simulink model "single_vector"  (R2018b)
settings: Solver=ode1  StartTime=0.0  StopTime=0.7  FixedStep=1e-6  RelTol=1e-4
undefined symbols (not defined in the file): Ba, DiscIntNeverNeededParam, flux, Ki, Kp, L, R, states, Ts, v
libraries: powerlib x4
settings Model: SimulationMode=accelerator  ExtModeTrigMode=oneshot  ExtModeArmWhenConnect=off  ExtModeAutoUpdateStatusClock=off  Creator=Administrador  LastModifiedBy=123
settings DataIOCC: SaveFormat=Array  SignalLoggingSaveFormat=ModelDataLogs  SignalLoggingName=sigsOut
settings OptimizationCC: BlockReduction=off  BooleanDataType=off  ExpressionDepthLimit=2147483647  InitFltsAndDblsToZero=on  LifeSpan=inf
settings DebuggingCC: SaveWithParameterizedLinksMsg=none  UnderspecifiedInitializationDetection=Classic  MergeDetectMultiDrivingBlocksExec=none  SignalResolutionControl=TryResolveAllWithWarning  MultiTaskDSMMsg=warning  MultiTaskCondExecSysMsg=none  FcnCallInpInsideContextMsg=warning  StateNameClashWarn=warning  LibraryContextMissingDiagnostic=none  SFUnexpectedBacktrackingDiag=warning  SFNoUnconditionalDefaultTransitionDiag=warning  SFExecutionAtInitializationDiag=none
settings HardwareCC: ProdBitPerPointer=32  ProdBitPerSizeT=32  ProdBitPerPtrDiffT=32  ProdLargestAtomicFloat=None  ProdIntDivRoundTo=Undefined  ProdEndianess=Unspecified  ProdWordSize=32  ProdHWDeviceType=32-bit Generic  TargetUnknown=on
settings ModelReferenceCC: PropagateSignalLabelsOutOfModel=off
settings SFSimCC: SimUseLocalCustomCode=off
settings RTWCC: RTWUseLocalCustomCode=off
settings CodeAppCC: StateflowObjectComments=on
settings GRTTargetCC: TargetFcnLib=ansi_tfl_tmw.mat  TargetLangStandard=C89/C90 (ANSI)  GeneratePreprocessorConditionals=Disable all  CombineOutputUpdateFcns=off  GRTInterface=on
settings ConfigComp: CovMetricSettings=dw  CovHtmlReporting=on  CovSaveCumulativeToWorkspaceVar=on  CovSaveSingleToWorkspaceVar=on  CovExternalEMLEnable=off  CovSFcnEnable=off

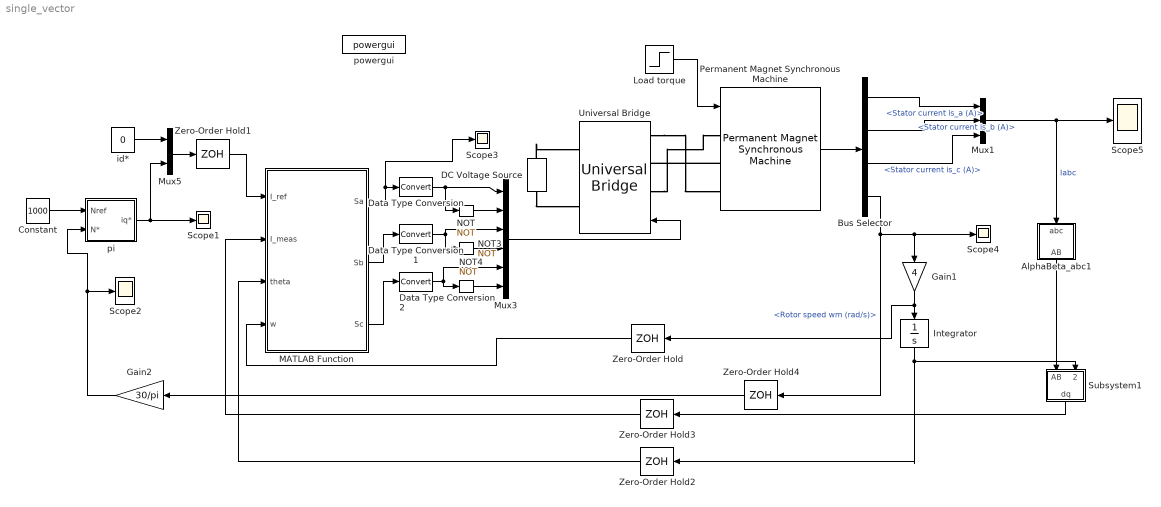
== system single_vector ==
  AlphaBeta_abc1 : Subsystem
  Bus Selector : BusSelector  OutputSignals=Stator current is_a (A),Stator current is_b (A),Stator current is_c (A),Rotor speed wm (rad/s)
  Constant : Constant  Value=1000
  DC Voltage Source : powerlib/Electrical Sources/DC Voltage Source  Amplitude=311  Measurements=None
      settings: SourceProductName=Simscape Electrical
  Data Type Conversion : DataTypeConversion
  Data Type Conversion1 : DataTypeConversion
  Data Type Conversion2 : DataTypeConversion
  Gain1 : Gain  Gain=4
  Gain2 : Gain  Gain=30/pi
  Integrator : Integrator
  Load torque : Step  Time=0.35  After=5  SampleTime=1e-6
  MATLAB Function : MATLAB Function  TreatAsAtomicUnit=on  SystemSampleTime=5e-6
  Mux1 : Mux  Inputs=3
  Mux3 : Mux  Inputs=6
  Mux5 : Mux  Inputs=2
  NOT : Logic  Operator=NOT  IconShape=distinctive  AllPortsSameDT=off  OutDataTypeStr=boolean
  NOT3 : Logic  Operator=NOT  IconShape=distinctive  AllPortsSameDT=off  OutDataTypeStr=boolean
  NOT4 : Logic  Operator=NOT  IconShape=distinctive  AllPortsSameDT=off  OutDataTypeStr=boolean
  Permanent Magnet Synchronous Machine : powerlib/Machines/Permanent Magnet Synchronous Machine  NbPhases=3  FluxDistribution=Sinusoidal  RotorType=Round  MechanicalLoad=Torque Tm  PresetModel=No  ShowDetailedParameters=on  MeasurementBus=off  Resistance=0.958  Inductance=8.5e-3  dqInductances=[5.25e-3,12e-3]  La=6e-3  MachineConstant=Flux linkage established by magnets (V.s)  Flux=0.1827  VoltageCst=132.5525  TorqueCst=1.0962  Flat=120  Mechanical=[0.003 0.008 4 0]  PolePairs=4  InitialConditions=[0,0, 0,0]  InitialConditions5ph=[0 0 0 0 0 0]  TsPowergui=0  TsBlock=-1  RefAngle=Aligned with phase A axis (original Park)
  Scope{1..5} (5 alike) : Scope
  Subsystem1 : Subsystem
  Universal Bridge : powerlib/Power Electronics/Universal Bridge  Arms=3  SnubberResistance=1e5  SnubberCapacitance=inf  Device=IGBT / Diodes  Ron=1e-3  Lon=0  ForwardVoltages="[  0  0  ]"  ForwardVoltage=0  GTOparameters=[ 10e-6 , 20e-6 ]  IGBTparameters=[ 1e-6 , 2e-6 ]  Measurements=None  Measurements_2=None  converterType=Rectifier
      settings: SourceProductName=Simscape Electrical
  Zero-Order Hold{,1..4} (5 alike) : ZeroOrderHold  SampleTime=5e-6
  id* : Constant  Value=0
  pi : Subsystem
  powergui : powerlib/powergui  Priority=1  SimulationMode=Discrete  SampleTime=1e-6  frequency=60  Iterations=50  frequencyindice=0  Pbase=100e6  ErrMax=1e-4  UnitsV=kV  UnitsW=MW  buscounter=0  FunctionMessages=off  echomessages=off  EnableUseOfTLC=off  CurrentSourceSwitches=off  DisableSnubberDevices=off  DisableRonSwitches=off  DisableVfSwitches=off  DisplayEquations=off  SolverType=Tustin  Interpol=off  ExternalGateDelay=off  methode=off  Ts=0  x0status=blocks  SPID=off  SwTol=0  HookPort=off  RestoreLinks=warning  ResistiveCurrentMeasurement=off  Frange=[0:2:500]  Ylog=off  Xlog=on  ShowGrid=off  save=off  variable=ZData  structure=ScopeData  ZoomFFT=off  StartTime=0.05  cycles=1  DisplayStyle=1  fundamental=50  FreqAxis=off  MaxFrequency=2000  frequencyindicesteady=1  RmsSteady=1  display=off
  wires:
  Mux1/1 -> Scope5/1, AlphaBeta_abc1/1(abc)  "Iabc"
  MATLAB Function/1(Sa) -> Scope3/1, Data Type Conversion/1
  NOT/1 -> Mux3/2
  MATLAB Function/2(Sb) -> Data Type Conversion1/1
  NOT3/1 -> Mux3/4
  MATLAB Function/3(Sc) -> Data Type Conversion2/1
  NOT4/1 -> Mux3/6
  Mux3/1 -> Universal Bridge/1
  Permanent Magnet Synchronous Machine/1 -> Bus Selector/1
  Bus Selector/1 -> Mux1/1  "<Stator current is_a (A)>"
  Bus Selector/2 -> Mux1/2  "<Stator current is_b (A)>"
  Bus Selector/3 -> Mux1/3  "<Stator current is_c (A)>"
  Constant/1 -> pi/1(Nref)
  Bus Selector/4 -> Gain1/1, Scope4/1, Zero-Order Hold4/1  "<Rotor speed wm (rad/s)>"
  AlphaBeta_abc1/1(AB) -> Subsystem1/1(AB)
  id*/1 -> Mux5/1
  pi/1(iq*) -> Scope1/1, Mux5/2
  Data Type Conversion/1 -> NOT/1, Mux3/1
  Data Type Conversion1/1 -> Mux3/3, NOT3/1
  Data Type Conversion2/1 -> Mux3/5, NOT4/1
  Mux5/1 -> Zero-Order Hold1/1
  Gain1/1 -> Zero-Order Hold/1, Integrator/1
  Integrator/1 -> Zero-Order Hold2/1, Subsystem1/2(theta)
  Load torque/1 -> Permanent Magnet Synchronous Machine/1
  Gain2/1 -> Scope2/1, pi/2(N*)
  Subsystem1/1(dq) -> Zero-Order Hold3/1
  Zero-Order Hold/1 -> MATLAB Function/4(w)
  Zero-Order Hold1/1 -> MATLAB Function/1(I_ref)
  Zero-Order Hold2/1 -> MATLAB Function/3(theta)
  Zero-Order Hold3/1 -> MATLAB Function/2(I_meas)
  Zero-Order Hold4/1 -> Gain2/1
  connections:
  DC Voltage Source/RConn1 -- Universal Bridge/RConn1
  DC Voltage Source/LConn1 -- Universal Bridge/RConn2
  Universal Bridge/LConn3 -- Permanent Magnet Synchronous Machine/LConn3
  Permanent Magnet Synchronous Machine/LConn2 -- Universal Bridge/LConn2
  Universal Bridge/LConn1 -- Permanent Magnet Synchronous Machine/LConn1

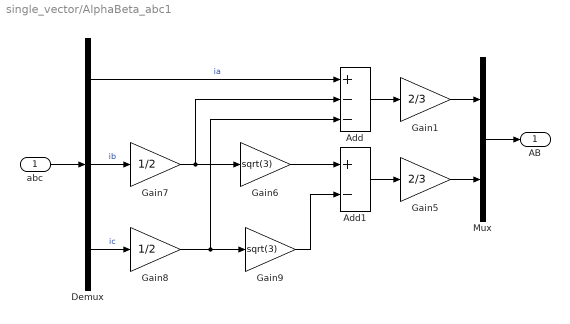
== system single_vector/AlphaBeta_abc1 ==
  abc : Inport
  Add : Sum  Inputs=+--
  Add1 : Sum  Inputs=+-
  Demux : Demux  Outputs=3
  Gain1 : Gain  Gain=2/3
  Gain5 : Gain  Gain=2/3
  Gain6 : Gain  Gain=sqrt(3)
  Gain7 : Gain  Gain=1/2
  Gain8 : Gain  Gain=1/2
  Gain9 : Gain  Gain=sqrt(3)
  Mux : Mux  Inputs=2
  AB : Outport
  wires:
  abc/1 -> Demux/1
  Demux/2 -> Gain7/1  "ib"
  Demux/3 -> Gain8/1  "ic"
  Add/1 -> Gain1/1
  Gain7/1 -> Gain6/1, Add/2
  Gain8/1 -> Gain9/1, Add/3
  Gain6/1 -> Add1/1
  Gain9/1 -> Add1/2
  Demux/1 -> Add/1  "ia"
  Add1/1 -> Gain5/1
  Gain1/1 -> Mux/1
  Gain5/1 -> Mux/2
  Mux/1 -> AB/1

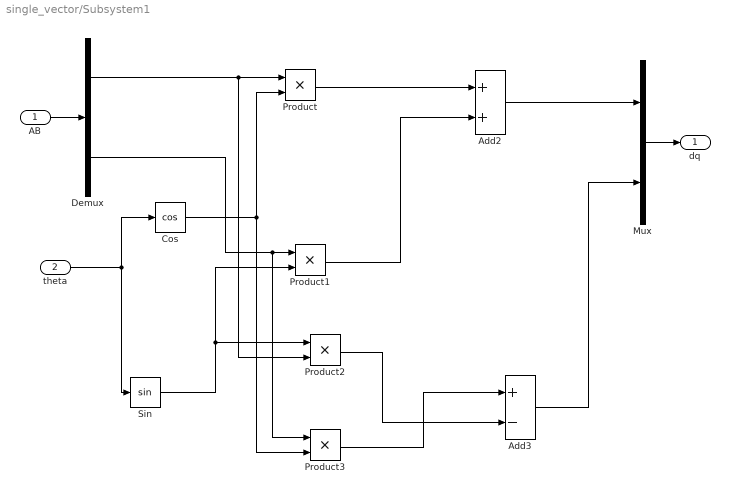
== system single_vector/Subsystem1 ==
  AB : Inport
  theta : Inport  Port=2
  Add2 : Sum
  Add3 : Sum  Inputs=+-
  Cos : Trigonometry  Operator=cos
  Demux : Demux  Outputs=2
  Mux : Mux  Inputs=2
  Product{,1..3} (4 alike) : Product
  Sin : Trigonometry
  dq : Outport
  wires:
  Product2/1 -> Add3/2
  Product/1 -> Add2/1
  theta/1 -> Sin/1, Cos/1
  Mux/1 -> dq/1
  AB/1 -> Demux/1
  Add3/1 -> Mux/2
  Add2/1 -> Mux/1
  Cos/1 -> Product3/2, Product/2
  Demux/2 -> Product1/1, Product3/1
  Demux/1 -> Product/1, Product2/2
  Product1/1 -> Add2/2
  Product3/1 -> Add3/1
  Sin/1 -> Product2/1, Product1/2

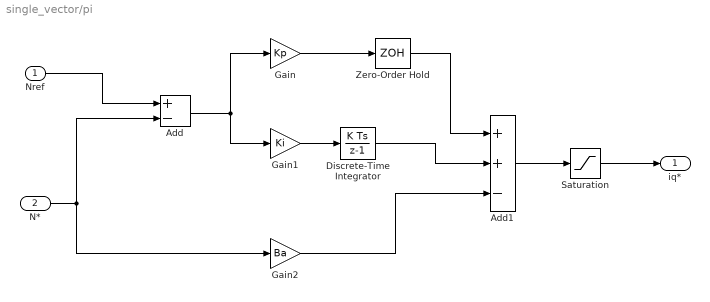
== system single_vector/pi ==
  Nref : Inport
  N* : Inport  Port=2
  Add : Sum  Inputs=+-
  Add1 : Sum  Inputs=++-
  Discrete-Time Integrator : DiscreteIntegrator  SampleTime=-1  ICPrevOutput=DiscIntNeverNeededParam  ICPrevScaledInput=DiscIntNeverNeededParam
  Gain : Gain  Gain=Kp
  Gain1 : Gain  Gain=Ki
  Gain2 : Gain  Gain=Ba
  Saturation : Saturate  UpperLimit=10  LowerLimit=-10
  Zero-Order Hold : ZeroOrderHold  SampleTime=-1
  iq* : Outport
  wires:
  Nref/1 -> Add/1
  N*/1 -> Gain2/1, Add/2
  Add/1 -> Gain1/1, Gain/1
  Gain/1 -> Zero-Order Hold/1
  Zero-Order Hold/1 -> Add1/1
  Gain1/1 -> Discrete-Time Integrator/1
  Discrete-Time Integrator/1 -> Add1/2
  Gain2/1 -> Add1/3
  Add1/1 -> Saturation/1
  Saturation/1 -> iq*/1

== matlab function single_vector/MATLAB Function ==
  data: I_ref input; Sa output; I_meas input; theta input; w input; Sb output; Sc output; R parameter; L parameter; Ts parameter; v parameter; states parameter; flux parameter
function [Sa,Sb,Sc] = control(I_ref,I_meas,theta,w,R, L, Ts, v, states, flux)

persistent x_old i_old 

if isempty(x_old), x_old = 1; end
if isempty(i_old), i_old = 0+1j*0; end
g = zeros(1,7);

ik_ref = I_ref(1) + 1j*I_ref(2);

ik = I_meas(1) + 1j*I_meas(2);
is = ik*exp(1j*theta);

% e = v(x_old) - L/Ts*is - (R - L/Ts)*i_old;
e = v(x_old) - R*(is+i_old)-L/Ts*(is-i_old);
en = e*exp(-1j*theta);

i_old = is;
for i = 1:7
    
    v_o1 = v(i)*exp(-1j*theta);
    
    % ik1 = (1 - R*Ts/L)*is + Ts/L*(v_o1 - e);
    ik_p = ik+Ts*(v_o1 - R*ik-w*L*ik-w*flux)/L;
    ik1 = ik_p+0.5*Ts*(-R)*(ik_p-ik)/L;
    u_ref = R*(ik_ref-ik1)*0.5+L*(ik_ref-ik1)/Ts+en;
   
    g(i) = abs(real(v_o1 - u_ref)) + abs(imag(v_o1 - u_ref));
    % g(i) = abs(real(is_ref - ik1)) + abs(imag(is_ref - ik1));
end
[~,x_opt] = min(g);

x_old = x_opt;

Sa = states(x_opt,1);
Sb = states(x_opt,2);
Sc = states(x_opt,3);
